simulink subsystem "subsys_force_2"  (R2021a)
settings: Solver=VariableStepAuto  StartTime=0.0  StopTime=10.0  RelTol=1e-3
values from neighbouring files (symbols this model uses):
  A_fe = [1.38863655835 325.252791044 4785.4211725 537388.603256 2685365.82642]    [coefficients.mat]
  A_fs = [0.0577985317911 23.8471094496 379.706147013 274153.88647]    [coefficients.mat]
  be = 13.029359254409743    (= 13.0293592544)    [Constante_L.m]    (also in Force.m; RunSimNL.m)
settings Model: Creator=antho  LastModifiedBy=antho

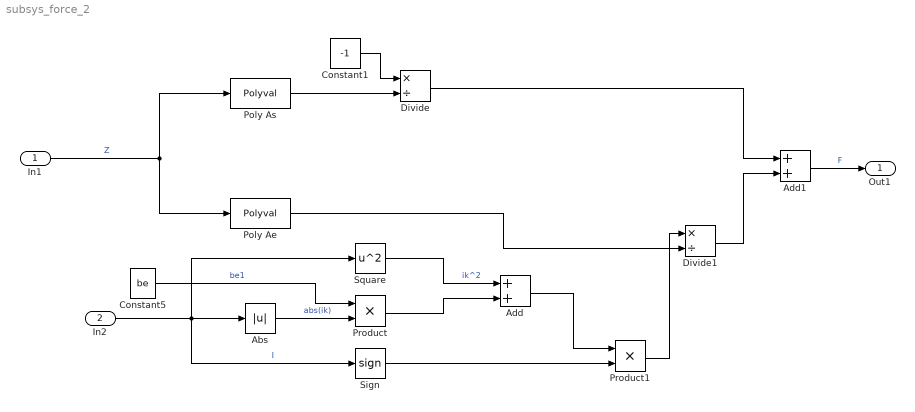
== system subsys_force_2 ==
  In1 : Inport
  In2 : Inport  Port=2
  Abs : Abs
  Add : Sum
  Add1 : Sum
  Constant1 : Constant  Value=-1
  Constant5 : Constant  Value=be
  Divide : Product  Inputs=*/
  Divide1 : Product  Inputs=*/
  Poly Ae : Polyval  Coefs=[A_fe(4) A_fe(3) A_fe(2) A_fe(1)]
  Poly As : Polyval  Coefs=[A_fs(4) A_fs(3) A_fs(2) A_fs(1)]
  Product : Product
  Product1 : Product
  Sign : Signum
  Square : Math  Operator=square  SaturateOnIntegerOverflow=on
  Out1 : Outport  SignalName=F
  wires:
  Add/1 -> Product1/1
  Product/1 -> Add/2
  Square/1 -> Add/1  "ik^2"
  Abs/1 -> Product/2  "abs(ik)"
  Sign/1 -> Product1/2
  Constant5/1 -> Product/1  "be1"
  In2/1 -> Square/1, Abs/1, Sign/1  "I"
  In1/1 -> Poly As/1, Poly Ae/1  "Z"
  Product1/1 -> Divide1/1
  Poly Ae/1 -> Divide1/2
  Poly As/1 -> Divide/2
  Constant1/1 -> Divide/1
  Divide1/1 -> Add1/2
  Divide/1 -> Add1/1
  Add1/1 -> Out1/1  "F"
